simulink model "BPSK"  (R2023b)
settings: Solver=VariableStepAuto  StartTime=0.0  StopTime=10.0  RelTol=1e-3
libraries: dspfdesign x1
settings Model: Creator=mluser  LastModifiedBy=mluser

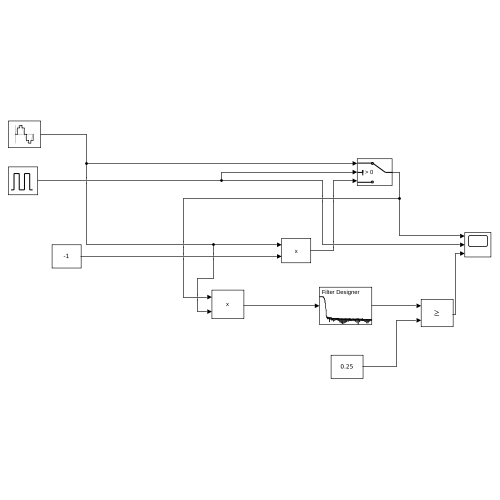
[thumbnail: Simulink's stored preview of the top-level diagram]
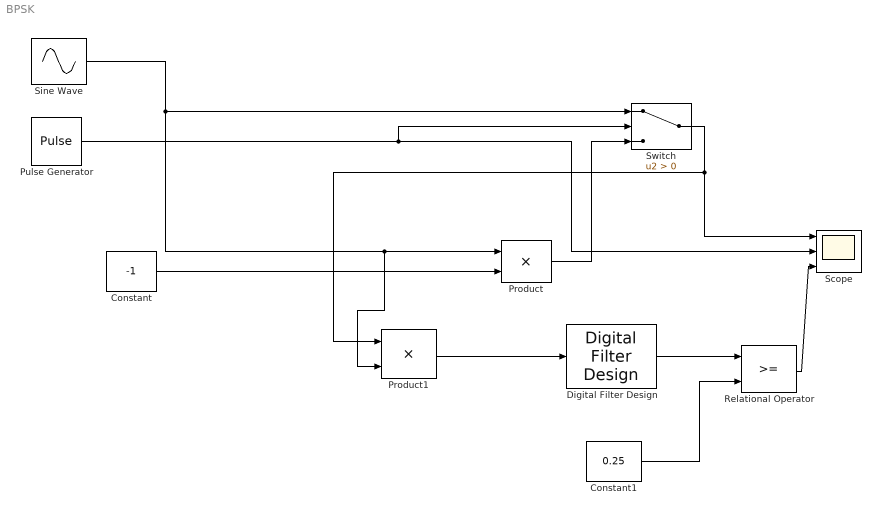
== system BPSK ==
  Constant : Constant  Value=-1
  Constant1 : Constant  Value=0.25
  Digital Filter Design : dspfdesign/Digital Filter Design  mwdsp_browser_bugfix_var=off
  Product : Product
  Product1 : Product
  Pulse Generator : DiscretePulseGenerator  PulseType=Time based  PulseWidth=50
  Relational Operator : RelationalOperator  OutDataTypeStr=boolean  RndMeth=Simplest  InputSameDT=off
  Scope : Scope  NumInputPorts=3
  Sine Wave : Sin  Frequency=2*pi*2  SampleTime=0.01
  Switch : Switch  Criteria=u2 > Threshold  SaturateOnIntegerOverflow=off  InputSameDT=off
  wires:
  Pulse Generator/1 -> Scope/2, Switch/2
  Sine Wave/1 -> Product1/2, Product/1, Switch/1
  Constant/1 -> Product/2
  Product/1 -> Switch/3
  Switch/1 -> Product1/1, Scope/1
  Product1/1 -> Digital Filter Design/1
  Digital Filter Design/1 -> Relational Operator/1
  Constant1/1 -> Relational Operator/2
  Relational Operator/1 -> Scope/3
